simulink model "Missile_Simulink_model"  (R2021a)
settings: Solver=ode4  StartTime=0.0  StopTime=10  FixedStep=Step_Size  RelTol=1e-3  EnableMultiTasking=on
InitFcn:
  | clc ;
  | clear all ;
  | close all ;
  | Missile_Data ;
  | Sim_Parameters ;
values from neighbouring files (symbols this model uses):
  D = 0.150    (= 0.15)    [Missile_Data.m]
  K_A = 0.0270    (= 0.027)    [Missile_Data.m]
  K_DC = 0.8443    [Missile_Data.m]
  K_p = 0.01    [Missile_Data.m]
  K_phi = 20.0    (= 20)    [Missile_Data.m]
  K_R = 0.0777    [Missile_Data.m]
  Mass = 30.0    (= 30)    [Missile_Data.m]
  Omega_i = -6.5208    [Missile_Data.m]
  S = ( pi / 4 ) * D^2    (= 0.0176714586764)    [Missile_Data.m]
  Tbl_ALPHAT = [ 0     4     8    12    16 ]    [Missile_Data.m]
  Tbl_CL_ALPHAT = [ -0.0988   -0.4859   -0.5870   -0.4802   -0.3334   -0.0210 ]    [Missile_Data.m]
  Tbl_CL_DEL_R = [ 5.2712    5.7640    6.1650    6.6234    7.1963    8.4110 ]    [Missile_Data.m]
  Tbl_CL_P = [ -17.9516  -19.6297  -20.9956  -22.5566  -24.5079  -28.6446 ]    [Missile_Data.m]
  Tbl_CM_0 = [ 0   -2.2250   -3.9280   -4.8580   -5.6940 ... (first row only)    [Missile_Data.m]
  Tbl_CM_DEL_P = [ -20.7182  -22.5631  -23.6059  -24.7632  -26.1269  -29.5646 ]    [Missile_Data.m]
  Tbl_CM_PHIT = [ 0   -0.0024   -0.0898   -0.2360   -0.3546 ... (first row only)    [Missile_Data.m]
  Tbl_CM_Q = [ -82.9643  -47.4409  -32.7732  -16.7304  -43.2010  -56.1499 ]    [Missile_Data.m]
  Tbl_CN_DEL_Y = [ -0.3616   -0.3938   -0.4120   -0.4322   -0.4560   -0.5160 ]    [Missile_Data.m]
  Tbl_CN_PHIT = [ 0    0.0040    0.0098    0.1116    0.3049 ... (first row only)    [Missile_Data.m]
  Tbl_CN_R = [ -82.9643  -47.4409  -32.7732  -16.7304  -43.2010  -56.1499 ]    [Missile_Data.m]
  Tbl_CX_0 = [ -0.3840   -0.3670   -0.3550   -0.3460   -0.3390   -0.3410 ]    [Missile_Data.m]
  Tbl_CX_ALPHAT = [ 0.0788    0.0752    0.0680    0.0573    0.0573    0.0573 ]    [Missile_Data.m]
  Tbl_CX_DEL_EFF = [ -16.8080  -17.8585  -18.9090  -19.9595  -20.4847  -23.1110 ]    [Missile_Data.m]
  Tbl_CY_DEL_Y = [ 5.3056    5.7754    6.0504    6.3484    6.6921    7.5745 ]    [Missile_Data.m]
  Tbl_CY_PHIT = [ 0    0.0070    0.0819    0.2313    0.2992 ... (first row only)    [Missile_Data.m]
  Tbl_CZ_0 = [ 0   -2.0680   -3.9700   -5.4250   -6.6810 ... (first row only)    [Missile_Data.m]
  Tbl_CZ_DEL_P = [ -5.3056   -5.7754   -6.0504   -6.3484   -6.6921   -7.5745 ]    [Missile_Data.m]
  Tbl_CZ_PHIT = [ 0    0.0089    0.1842    0.3041    0.2039 ... (first row only)    [Missile_Data.m]
  Tbl_MACH = [ 0.2    0.3    0.4    0.5    0.6    0.7 ]    [Missile_Data.m]
  UNIT_GRAV = 9.81    [Sim_Parameters.m]
  Wn_Act = 25.0 * 2 * pi    (= 157.079632679)    [Missile_Data.m]
  XCG = 0.809    [Missile_Data.m]
  XREF = 0.809    [Missile_Data.m]
  Zeta_Act = 0.707    [Missile_Data.m]
libraries: simulink_extras x6, aerolibtransform2 x4, aerolibasang x3, aerolibconvert2 x2, shared6dof x1, aerolibatmos2 x1
(part 1 of 2)
settings Model: Creator=e803534  LastModifiedBy=s347520
settings SolverCC: AlgebraicLoopSolver=TrustRegion
settings DataIOCC: ReturnWorkspaceOutputs=off
settings OptimizationCC: LifeSpan=inf
settings DebuggingCC: UnconnectedInputMsg=none  UnconnectedOutputMsg=none  UnconnectedLineMsg=none  SFUnexpectedBacktrackingDiag=warning  SFNoUnconditionalDefaultTransitionDiag=warning  SFMachineParentedDataDiag=warning  ArithmeticOperatorsInVariantConditions=warning
settings SFSimCC: SimUseLocalCustomCode=off  CustomCodeUndefinedFunction=UseInterfaceOnly
settings RTWCC: RTWUseLocalCustomCode=off
settings CodeAppCC: StateflowObjectComments=on
settings GRTTargetCC: TargetLangStandard=C89/C90 (ANSI)
settings ConfigComp: CovMetricSettings=dw  CovSaveCumulativeToWorkspaceVar=on  CovSaveSingleToWorkspaceVar=on  CovExternalEMLEnable=off

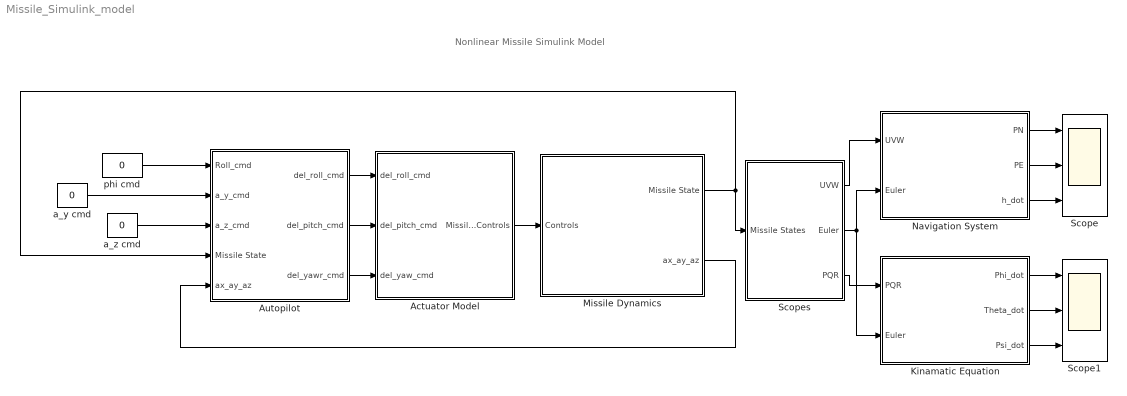
== system Missile_Simulink_model ==
  note: Nonlinear Missile Simulink Model
  Actuator Model : Subsystem
  "Autopilot " : Subsystem
  Kinamatic Equation : Subsystem
  Missile Dynamics : Subsystem
  Navigation System : Subsystem
  Scope : Scope  NumInputPorts=3
  Scope1 : Scope  NumInputPorts=3
  Scopes : Subsystem
  a_y cmd : Constant  Value=0
  a_z cmd : Constant  Value=0
  phi cmd : Constant  Value=0
  wires:
  "Autopilot "/2(del_pitch_cmd) -> Actuator Model/2(del_pitch_cmd)
  "Autopilot "/1(del_roll_cmd) -> Actuator Model/1(del_roll_cmd)
  "Autopilot "/3(del_yawr_cmd) -> Actuator Model/3(del_yaw_cmd)
  Missile Dynamics/1(Missile State) -> "Autopilot "/4(Missile State), Scopes/1(Missile States)
  a_z cmd/1 -> "Autopilot "/3(a_z_cmd)
  phi cmd/1 -> "Autopilot "/1(Roll_cmd)
  a_y cmd/1 -> "Autopilot "/2(a_y_cmd)
  Missile Dynamics/2(ax_ay_az) -> "Autopilot "/5(ax_ay_az)
  Actuator Model/1(Missile_Controls) -> Missile Dynamics/1(Controls)
  Scopes/1(UVW) -> Navigation System/1(UVW)
  Scopes/2(Euler) -> Kinamatic Equation/2(Euler), Navigation System/2(Euler)
  Navigation System/1(PN) -> Scope/1
  Navigation System/2(PE) -> Scope/2
  Navigation System/3(h_dot) -> Scope/3
  Scopes/3(PQR) -> Kinamatic Equation/1(PQR)
  Kinamatic Equation/1(Phi_dot) -> Scope1/1
  Kinamatic Equation/2(Theta_dot) -> Scope1/2
  Kinamatic Equation/3(Psi_dot) -> Scope1/3

== system Missile_Simulink_model/Actuator Model ==
  note: Actuator Model
  del_roll_cmd : Inport
  del_pitch_cmd : Inport  Port=2
  del_yaw_cmd : Inport  Port=3
  Mux : Mux  Inputs=3
  Saturation : Saturate  UpperLimit=10  LowerLimit=-10
  Saturation1 : Saturate  UpperLimit=10  LowerLimit=-10
  Saturation2 : Saturate  UpperLimit=10  LowerLimit=-10
  Transfer Fcn : TransferFcn  Numerator=[Wn_Act^2]  Denominator=[1 2*Zeta_Act*Wn_Act Wn_Act^2]
  Transfer Fcn1 : TransferFcn  Numerator=[Wn_Act^2]  Denominator=[1 2*Zeta_Act*Wn_Act Wn_Act^2]
  Transfer Fcn2 : TransferFcn  Numerator=[Wn_Act^2]  Denominator=[1 2*Zeta_Act*Wn_Act Wn_Act^2]
  Missile_Controls : Outport  VectorParamsAs1DForOutWhenUnconnected=off
  wires:
  del_roll_cmd/1 -> Transfer Fcn/1
  Mux/1 -> Missile_Controls/1
  del_yaw_cmd/1 -> Transfer Fcn2/1
  del_pitch_cmd/1 -> Transfer Fcn1/1
  Transfer Fcn/1 -> Saturation/1
  Transfer Fcn1/1 -> Saturation1/1
  Transfer Fcn2/1 -> Saturation2/1
  Saturation/1 -> Mux/1
  Saturation2/1 -> Mux/3
  Saturation1/1 -> Mux/2

== system Missile_Simulink_model/Autopilot  ==
  note: Autopilot
  Roll_cmd : Inport
  a_y_cmd : Inport  Port=2
  a_z_cmd : Inport  Port=3
  Missile State : Inport  Port=4
  ax_ay_az : Inport  Port=5
  Mux : Mux  Inputs=3
  Pitch Control : Subsystem
  Roll Control : Subsystem
  Scope : Scope
  Yaw Control : Subsystem
  del_roll_cmd : Outport  VectorParamsAs1DForOutWhenUnconnected=off
  del_pitch_cmd : Outport  Port=2  VectorParamsAs1DForOutWhenUnconnected=off
  del_yawr_cmd : Outport  Port=3  VectorParamsAs1DForOutWhenUnconnected=off
  wires:
  Missile State/1 -> Pitch Control/2(Missile_State), Yaw Control/1(Missile_State), Roll Control/2(Missile_State)
  a_z_cmd/1 -> Pitch Control/1(a_z_cmd)
  Pitch Control/1(del_p_cmd) -> Mux/2, del_pitch_cmd/1
  Roll_cmd/1 -> Roll Control/1(Roll_cmd)
  Roll Control/1(del_r_cmd) -> Mux/1, del_roll_cmd/1
  a_y_cmd/1 -> Yaw Control/2("a_y_cmd ")
  Yaw Control/1(del_r_cmd) -> Mux/3, del_yawr_cmd/1
  ax_ay_az/1 -> Pitch Control/3(ax_ay_az), Yaw Control/3(ax_ay_az)
  Mux/1 -> Scope/1

== system Missile_Simulink_model/Kinamatic Equation ==
  PQR : Inport
  Euler : Inport  Port=2
  Demux : Demux  Outputs=3
  Demux2 : Demux  Outputs=3
  MATLAB Function4 : MATLAB Function  TreatAsAtomicUnit=on
  Phi_dot : Outport
  Theta_dot : Outport  Port=2
  Psi_dot : Outport  Port=3
  wires:
  PQR/1 -> Demux2/1
  Euler/1 -> Demux/1
  Demux/1 -> MATLAB Function4/4(phi)
  Demux/2 -> MATLAB Function4/5(theta)
  Demux/3 -> MATLAB Function4/6(psi)
  Demux2/1 -> MATLAB Function4/1(p)
  Demux2/2 -> MATLAB Function4/2(q)
  Demux2/3 -> MATLAB Function4/3(r)
  MATLAB Function4/1(Phi_dot) -> Phi_dot/1
  MATLAB Function4/2(Theta_dot) -> Theta_dot/1
  MATLAB Function4/3(Psi_dot) -> Psi_dot/1

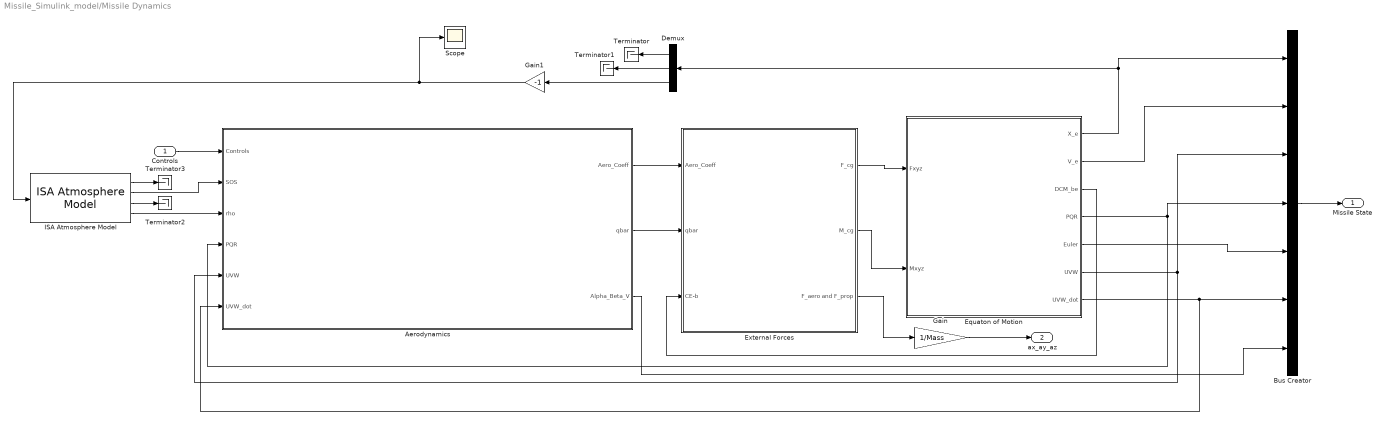
== system Missile_Simulink_model/Missile Dynamics ==
  Controls : Inport
  Aerodynamics : Subsystem
  Bus Creator : BusCreator  Inputs=7
  Demux : Demux  Outputs=3
  Equaton of Motion : Subsystem
  External Forces : Subsystem
  Gain : Gain  Gain=1/Mass
  Gain1 : Gain  Gain=-1
  ISA Atmosphere Model : aerolibatmos2/ISA Atmosphere Model  custom=off  g=9.80665  gamma=1.4  R=287.0531  L=0.0065  h_trop=11000  h_strat=20000  rho0=1.225  P0=101325  T0=288.15  h0=0
  Scope : Scope
  Terminator{,1..3} (4 alike) : Terminator
  Missile State : Outport  VectorParamsAs1DForOutWhenUnconnected=off
  ax_ay_az : Outport  Port=2  VectorParamsAs1DForOutWhenUnconnected=off
  wires:
  Bus Creator/1 -> Missile State/1
  External Forces/3(F_aero and F_prop) -> Gain/1
  Gain/1 -> ax_ay_az/1
  Controls/1 -> Aerodynamics/1(Controls)
  ISA Atmosphere Model/2 -> Aerodynamics/2(SOS)
  ISA Atmosphere Model/4 -> Aerodynamics/3(rho)
  Aerodynamics/1(Aero_Coeff) -> External Forces/1(Aero_Coeff)
  Aerodynamics/2(qbar) -> External Forces/2(qbar)
  Aerodynamics/3(Alpha_Beta_V) -> Bus Creator/7
  Equaton of Motion/4(PQR) -> Aerodynamics/4(PQR), Bus Creator/4
  Equaton of Motion/6(UVW) -> Bus Creator/3, Aerodynamics/5(UVW)
  Equaton of Motion/2(V_e) -> Bus Creator/2
  Equaton of Motion/1(X_e) -> Demux/1, Bus Creator/1
  Equaton of Motion/7(UVW_dot) -> Aerodynamics/6(UVW_dot), Bus Creator/6
  External Forces/1(F_cg) -> Equaton of Motion/1(Fxyz)
  External Forces/2(M_cg) -> Equaton of Motion/2(Mxyz)
  Equaton of Motion/3(DCM_be) -> External Forces/3(CE-b)
  Equaton of Motion/5(Euler) -> Bus Creator/5
  Demux/3 -> Gain1/1
  Gain1/1 -> Scope/1, ISA Atmosphere Model/1
  Demux/1 -> Terminator/1
  Demux/2 -> Terminator1/1
  ISA Atmosphere Model/3 -> Terminator2/1
  ISA Atmosphere Model/1 -> Terminator3/1

== system Missile_Simulink_model/Navigation System ==
  note: h
  note: PE
  note: PN
  note: VD
  note: VE
  note: VN
  UVW : Inport
  Euler : Inport  Port=2
  Demux : Demux  Outputs=3
  Demux1 : Demux  Outputs=3
  Demux2 : Demux  Outputs=3
  Gain : Gain  Gain=-1
  Integrator1 : Integrator
  Integrator2 : Integrator
  Integrator3 : Integrator
  MATLAB Function4 : MATLAB Function  TreatAsAtomicUnit=on
  Matrix Multiply2 : Product  Multiplication=Matrix(*)
  Mux : Mux  Inputs=3
  PN : Outport
  PE : Outport  Port=2
  h_dot : Outport  Port=3
  wires:
  Demux1/2 -> Integrator2/1
  Gain/1 -> Integrator3/1
  Integrator1/1 -> PN/1
  Mux/1 -> Matrix Multiply2/2
  Demux/2 -> MATLAB Function4/2(theta)
  Demux/3 -> MATLAB Function4/3(psi)
  Demux/1 -> MATLAB Function4/1(phi)
  Integrator2/1 -> PE/1
  Integrator3/1 -> h_dot/1
  Demux1/3 -> Gain/1
  Demux1/1 -> Integrator1/1
  Demux2/1 -> Mux/1
  Demux2/2 -> Mux/2
  Demux2/3 -> Mux/3
  Euler/1 -> Demux/1
  UVW/1 -> Demux2/1
  MATLAB Function4/1(C1) -> Matrix Multiply2/1
  Matrix Multiply2/1 -> Demux1/1

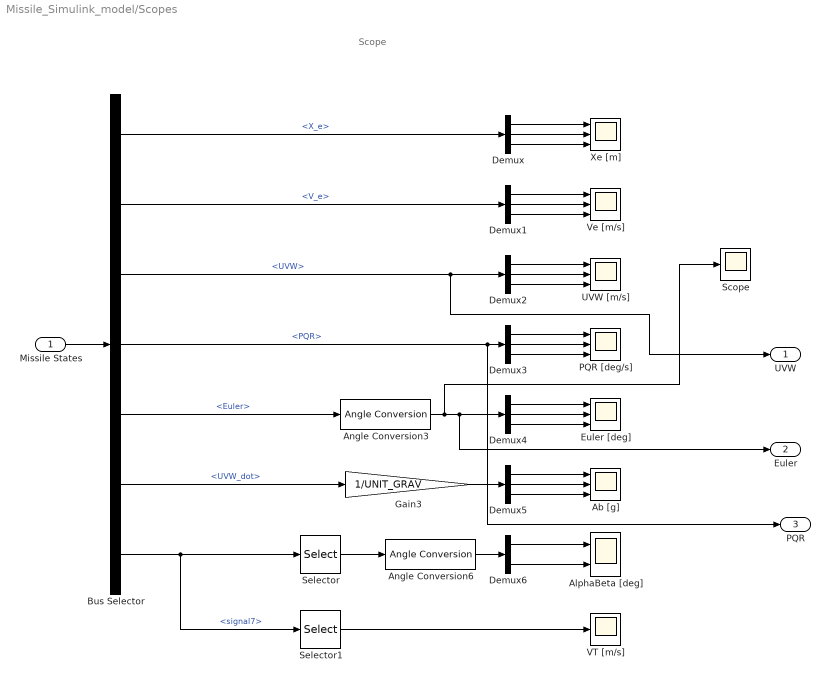
== system Missile_Simulink_model/Scopes ==
  note: Scope
  Missile States : Inport
  Ab [g] : Scope  NumInputPorts=3
  AlphaBeta [deg] : Scope  NumInputPorts=2
  Angle Conversion3 : aerolibconvert2/Angle Conversion  IU=rad  OU=deg
  Angle Conversion6 : aerolibconvert2/Angle Conversion  IU=rad  OU=deg
  Bus Selector : BusSelector  OutputSignals=X_e,V_e,UVW,PQR,Euler,UVW_dot,signal7
  Demux{,1..5} (6 alike) : Demux  Outputs=3
  Demux6 : Demux  Outputs=2
  Euler [deg] : Scope  NumInputPorts=3
  Gain3 : Gain  Gain=1/UNIT_GRAV
  PQR [deg/s] : Scope  NumInputPorts=3
  Scope : Scope
  Selector : Selector  InputPortWidth=3  IndexOptions=Index vector (dialog)  Indices=[1 2]  OutputSizes=1
  Selector1 : Selector  InputPortWidth=3  IndexOptions=Index vector (dialog)  Indices=[3]  OutputSizes=1
  UVW [m/s] : Scope  NumInputPorts=3
  VT [m/s] : Scope
  Ve [m/s] : Scope  NumInputPorts=3
  Xe [m] : Scope  NumInputPorts=3
  UVW : Outport
  Euler : Outport  Port=2
  PQR : Outport  Port=3
  wires:
  Missile States/1 -> Bus Selector/1
  Bus Selector/1 -> Demux/1  "<X_e>"
  Bus Selector/2 -> Demux1/1  "<V_e>"
  Bus Selector/3 -> UVW/1, Demux2/1  "<UVW>"
  Bus Selector/4 -> PQR/1, Demux3/1  "<PQR>"
  Bus Selector/5 -> Angle Conversion3/1  "<Euler>"
  Bus Selector/6 -> Gain3/1  "<UVW_dot>"
  Angle Conversion3/1 -> Scope/1, Euler/1, Demux4/1
  Selector1/1 -> VT [m/s]/1
  Gain3/1 -> Demux5/1
  Demux/1 -> Xe [m]/1
  Demux/2 -> Xe [m]/2
  Demux/3 -> Xe [m]/3
  Demux1/1 -> Ve [m/s]/1
  Demux1/2 -> Ve [m/s]/2
  Demux1/3 -> Ve [m/s]/3
  Demux2/1 -> UVW [m/s]/1
  Demux2/2 -> UVW [m/s]/2
  Demux2/3 -> UVW [m/s]/3
  Demux3/1 -> PQR [deg/s]/1
  Demux3/2 -> PQR [deg/s]/2
  Demux3/3 -> PQR [deg/s]/3
  Demux4/1 -> Euler [deg]/1
  Demux4/2 -> Euler [deg]/2
  Demux4/3 -> Euler [deg]/3
  Demux5/1 -> Ab [g]/1
  Demux5/2 -> Ab [g]/2
  Demux5/3 -> Ab [g]/3
  Demux6/2 -> AlphaBeta [deg]/2
  Demux6/1 -> AlphaBeta [deg]/1
  Angle Conversion6/1 -> Demux6/1
  Bus Selector/7 -> Selector1/1, Selector/1  "<signal7>"
  Selector/1 -> Angle Conversion6/1

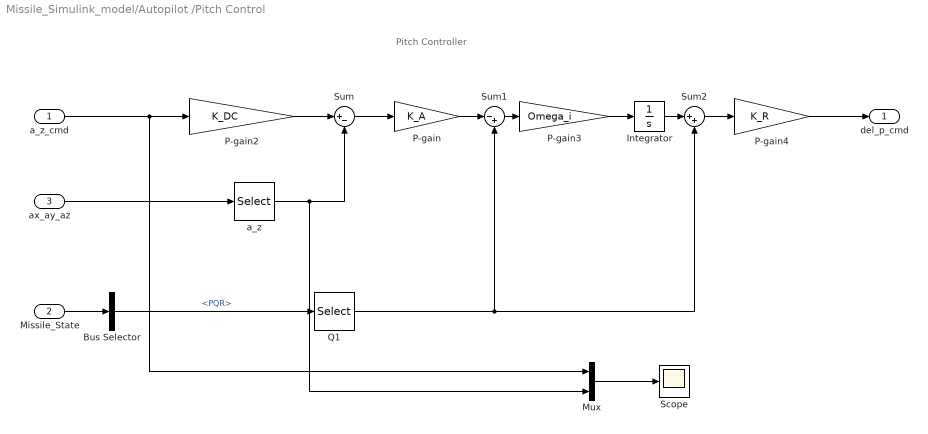
== system Missile_Simulink_model/Autopilot /Pitch Control ==
  note: Pitch Controller
  a_z_cmd : Inport
  Missile_State : Inport  Port=2
  ax_ay_az : Inport  Port=3
  Bus Selector : BusSelector  OutputSignals=PQR
  Integrator : Integrator
  Mux : Mux  Inputs=2
  P-gain : Gain  Gain=K_A
  P-gain2 : Gain  Gain=K_DC
  P-gain3 : Gain  Gain=Omega_i
  P-gain4 : Gain  Gain=K_R
  Q1 : Selector  InputPortWidth=3  IndexOptions=Index vector (dialog)  Indices=[2]  OutputSizes=1
  Scope : Scope
  Sum : Sum  Inputs=|+-
  Sum1 : Sum  Inputs=|-+
  Sum2 : Sum  Inputs=|++
  a_z : Selector  InputPortWidth=3  IndexOptions=Index vector (dialog)  Indices=[3]  OutputSizes=1
  del_p_cmd : Outport  VectorParamsAs1DForOutWhenUnconnected=off
  wires:
  Missile_State/1 -> Bus Selector/1
  P-gain/1 -> Sum1/1
  a_z/1 -> Mux/2, Sum/2
  ax_ay_az/1 -> a_z/1
  P-gain4/1 -> del_p_cmd/1
  Bus Selector/1 -> Q1/1  "<PQR>"
  Q1/1 -> Sum2/2, Sum1/2
  a_z_cmd/1 -> Mux/1, P-gain2/1
  Sum1/1 -> P-gain3/1
  Sum/1 -> P-gain/1
  P-gain2/1 -> Sum/1
  P-gain3/1 -> Integrator/1
  Sum2/1 -> P-gain4/1
  Mux/1 -> Scope/1
  Integrator/1 -> Sum2/1

== system Missile_Simulink_model/Autopilot /Roll Control ==
  note: Roll Controller
  Roll_cmd : Inport
  Missile_State : Inport  Port=2
  Bus Selector : BusSelector  OutputSignals=Euler,PQR
  P : Selector  InputPortWidth=3  IndexOptions=Index vector (dialog)  Indices=[1]  OutputSizes=1
  P-gain2 : Gain  Gain=K_phi
  P-gain3 : Gain  Gain=K_p
  PHI : Selector  InputPortWidth=3  IndexOptions=Index vector (dialog)  Indices=[1]  OutputSizes=1
  Sum : Sum  Inputs=|+-
  Sum2 : Sum  Inputs=|+-
  del_r_cmd : Outport  VectorParamsAs1DForOutWhenUnconnected=off
  wires:
  P-gain2/1 -> Sum2/1
  Missile_State/1 -> Bus Selector/1
  Bus Selector/2 -> P/1  "<PQR>"
  P/1 -> Sum2/2
  PHI/1 -> Sum/2
  Roll_cmd/1 -> Sum/1
  Sum2/1 -> P-gain3/1
  Sum/1 -> P-gain2/1
  Bus Selector/1 -> PHI/1  "<Euler>"
  P-gain3/1 -> del_r_cmd/1

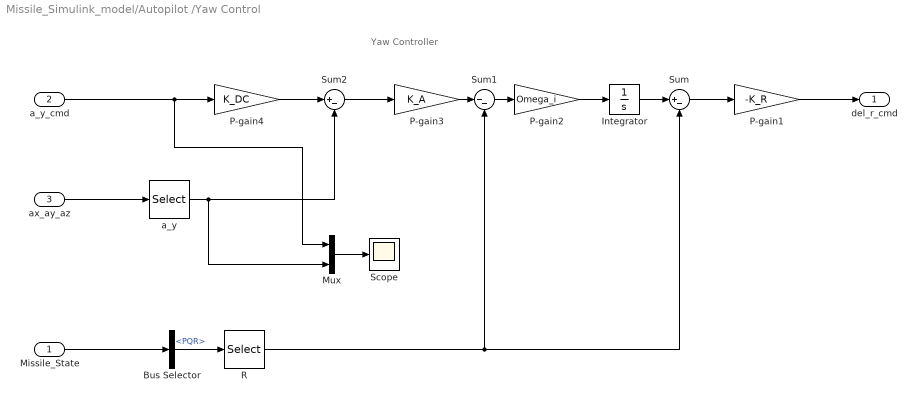
== system Missile_Simulink_model/Autopilot /Yaw Control ==
  note: Yaw Controller
  Missile_State : Inport
  "a_y_cmd " : Inport  Port=2
  ax_ay_az : Inport  Port=3
  Bus Selector : BusSelector  OutputSignals=PQR
  Integrator : Integrator
  Mux : Mux  Inputs=2
  P-gain1 : Gain  Gain=-K_R
  P-gain2 : Gain  Gain=Omega_i
  P-gain3 : Gain  Gain=K_A
  P-gain4 : Gain  Gain=K_DC
  R : Selector  InputPortWidth=3  IndexOptions=Index vector (dialog)  Indices=[3]  OutputSizes=1
  Scope : Scope
  Sum : Sum  Inputs=|+-
  Sum1 : Sum  Inputs=|--
  Sum2 : Sum  Inputs=|+-
  a_y : Selector  InputPortWidth=3  IndexOptions=Index vector (dialog)  Indices=[2]  OutputSizes=1
  del_r_cmd : Outport  VectorParamsAs1DForOutWhenUnconnected=off
  wires:
  ax_ay_az/1 -> a_y/1
  P-gain3/1 -> Sum1/1
  R/1 -> Sum1/2, Sum/2
  Sum2/1 -> P-gain3/1
  P-gain1/1 -> del_r_cmd/1
  Sum1/1 -> P-gain2/1
  Bus Selector/1 -> R/1  "<PQR>"
  "a_y_cmd "/1 -> Mux/1, P-gain4/1
  Sum/1 -> P-gain1/1
  Integrator/1 -> Sum/1
  Missile_State/1 -> Bus Selector/1
  P-gain2/1 -> Integrator/1
  a_y/1 -> Mux/2, Sum2/2
  Mux/1 -> Scope/1
  P-gain4/1 -> Sum2/1

== system Missile_Simulink_model/Missile Dynamics/Aerodynamics ==
  Controls : Inport
  SOS : Inport  Port=2
  rho : Inport  Port=3
  PQR : Inport  Port=4
  UVW : Inport  Port=5
  UVW_dot : Inport  Port=6
  Aerodynamic Coefficient : Subsystem
  Ground : Ground
  Ground1 : Ground
  Wind-axes Velocitie : Subsystem  AncestorBlock=UAS_Model_library/External Forces/Aerodynamics/Wind-axes Velocitie
  Aero_Coeff : Outport  VectorParamsAs1DForOutWhenUnconnected=off
  qbar : Outport  Port=2  VectorParamsAs1DForOutWhenUnconnected=off
  Alpha_Beta_V : Outport  Port=3  VectorParamsAs1DForOutWhenUnconnected=off
  wires:
  rho/1 -> Wind-axes Velocitie/4(Rho)
  UVW/1 -> Wind-axes Velocitie/1(UVW)
  Wind-axes Velocitie/1(Alpha_Beta_V) -> Alpha_Beta_V/1, Aerodynamic Coefficient/3(Alpha_Beta_V1), Aerodynamic Coefficient/2(Alpha_Beta_V)
  Wind-axes Velocitie/2(Mach) -> Aerodynamic Coefficient/4(Mach Number)
  Ground1/1 -> Wind-axes Velocitie/2(Wind_Vel)
  Ground/1 -> Wind-axes Velocitie/7(Wind_Rate)
  Controls/1 -> Aerodynamic Coefficient/1(Control)
  PQR/1 -> Aerodynamic Coefficient/5(PQR), Wind-axes Velocitie/6(PQR)
  Wind-axes Velocitie/3(qbar) -> qbar/1
  UVW_dot/1 -> Wind-axes Velocitie/5(UVW_dot)
  Aerodynamic Coefficient/1(Aero_Coeff) -> Aero_Coeff/1
  SOS/1 -> Wind-axes Velocitie/3(SoS)

== system Missile_Simulink_model/Missile Dynamics/Equaton of Motion ==
  Fxyz : Inport
  Mxyz : Inport  Port=2
  Equation of mortion : Subsystem
  Terminator2 : Terminator
  X_e : Outport  VectorParamsAs1DForOutWhenUnconnected=off
  V_e : Outport  Port=2  VectorParamsAs1DForOutWhenUnconnected=off
  DCM_be : Outport  Port=3  VectorParamsAs1DForOutWhenUnconnected=off
  PQR : Outport  Port=4  VectorParamsAs1DForOutWhenUnconnected=off
  Euler : Outport  Port=5  VectorParamsAs1DForOutWhenUnconnected=off
  UVW : Outport  Port=6  VectorParamsAs1DForOutWhenUnconnected=off
  UVW_dot : Outport  Port=7  VectorParamsAs1DForOutWhenUnconnected=off
  wires:
  Fxyz/1 -> Equation of mortion/1(Forces)
  Mxyz/1 -> Equation of mortion/2(Moments)
  Equation of mortion/1(V_e) -> V_e/1
  Equation of mortion/2(X_e) -> X_e/1
  Equation of mortion/3(Euler) -> Euler/1
  Equation of mortion/4(DCM) -> DCM_be/1
  Equation of mortion/5(UVW) -> UVW/1
  Equation of mortion/6(PQR) -> PQR/1
  Equation of mortion/7(pdot,qdot,rdot) -> Terminator2/1
  Equation of mortion/8(UVW_dot) -> UVW_dot/1

== system Missile_Simulink_model/Missile Dynamics/External Forces ==
  Aero_Coeff : Inport
  qbar : Inport  Port=2
  CE-b : Inport  Port=3
  Add : Sum
  Aerodynamic Force & Moment : Subsystem  AncestorBlock=UAS_Model_library/External Forces/Aerodynamics/Aerodynamic Force & Moment
  Propulsive Force & Moment : Subsystem  AncestorBlock=UAS_Model_library/External Forces/Propulsive/Propulsive Force & Moment
  Total Force & Moment : Subsystem  AncestorBlock=UAS_Model_library/External Forces/Total Force & Moment
  F_cg : Outport  VectorParamsAs1DForOutWhenUnconnected=off
  M_cg : Outport  Port=2  VectorParamsAs1DForOutWhenUnconnected=off
  F_aero and F_prop : Outport  Port=3  VectorParamsAs1DForOutWhenUnconnected=off
  wires:
  Total Force & Moment/2(M_cg) -> M_cg/1
  Aerodynamic Force & Moment/2(M_aero) -> Total Force & Moment/2(M_aero)
  Propulsive Force & Moment/2(M_prop) -> Total Force & Moment/4(M_prop)
  Total Force & Moment/1(F_cg) -> F_cg/1
  Aerodynamic Force & Moment/1(F_aero) -> Add/1, Total Force & Moment/1(F_aero)
  Propulsive Force & Moment/1(F_prop) -> Add/2, Total Force & Moment/3(F_prop)
  qbar/1 -> Aerodynamic Force & Moment/2(qbar)
  Aero_Coeff/1 -> Aerodynamic Force & Moment/1(Aero_Coeff)
  Add/1 -> F_aero and F_prop/1
  CE-b/1 -> Total Force & Moment/5("cE-B ")

== system Missile_Simulink_model/Missile Dynamics/Aerodynamics/Aerodynamic Coefficient ==
  Control : Inport
  Alpha_Beta_V : Inport  Port=2
  Alpha_Beta_V1 : Inport  Port=3
  Mach Number : Inport  Port=4
  PQR : Inport  Port=5
  Aerodynamics : Subsystem
  delta_eff : Subsystem
  total angle of AoA and Roll : Subsystem
  Aero_Coeff : Outport  VectorParamsAs1DForOutWhenUnconnected=off
  wires:
  total angle of AoA and Roll/1(alpha_t) -> Aerodynamics/4(alpha_t)
  Alpha_Beta_V/1 -> Aerodynamics/6(alpha_beta_V)
  total angle of AoA and Roll/2(phi_t) -> Aerodynamics/5(phi_t)
  delta_eff/1(delta_eff) -> Aerodynamics/2(delta_eff)
  Control/1 -> Aerodynamics/3(control inputs), delta_eff/1(controll)
  Aerodynamics/1(Aero_Coeff) -> Aero_Coeff/1
  Alpha_Beta_V1/1 -> total angle of AoA and Roll/1(alpha_beta_V)
  Mach Number/1 -> Aerodynamics/1(Mach Number)
  PQR/1 -> Aerodynamics/7(PQR)

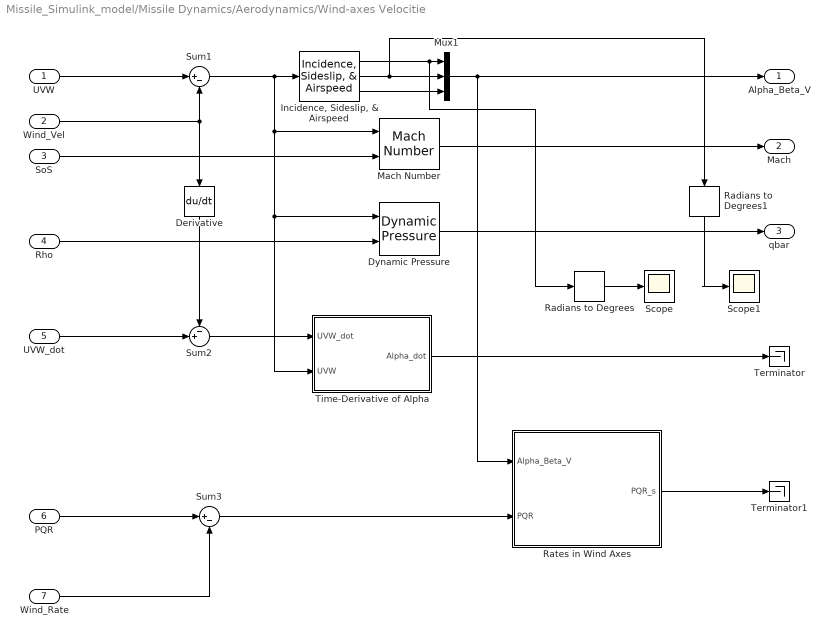
== system Missile_Simulink_model/Missile Dynamics/Aerodynamics/Wind-axes Velocitie ==
  UVW : Inport
  Wind_Vel : Inport  Port=2
  SoS : Inport  Port=3
  Rho : Inport  Port=4
  UVW_dot : Inport  Port=5
  PQR : Inport  Port=6
  Wind_Rate : Inport  Port=7
  Derivative : Derivative
  Dynamic Pressure : aerolibasang/Dynamic Pressure
  "Incidence, Sideslip, & Airspeed" : aerolibasang/Incidence, Sideslip, & Airspeed
  Mach Number : aerolibasang/Mach Number
      settings: SourceProductBaseCode=AE
  Mux1 : Mux  Inputs=3
  Radians to Degrees : simulink_extras/Transformations/Radians to Degrees
  Radians to Degrees1 : simulink_extras/Transformations/Radians to Degrees
  Rates in Wind Axes : Subsystem
  Scope : Scope
  Scope1 : Scope
  Sum1 : Sum  Inputs=|+-  InputSameDT=on  SaturateOnIntegerOverflow=on  OutDataTypeStr=Inherit: Same as first input
  Sum2 : Sum  Inputs=-+|  InputSameDT=on  SaturateOnIntegerOverflow=on  OutDataTypeStr=Inherit: Same as first input
  Sum3 : Sum  Inputs=|+-  InputSameDT=on  SaturateOnIntegerOverflow=on  OutDataTypeStr=Inherit: Same as first input
  Terminator : Terminator
  Terminator1 : Terminator
  Time-Derivative of Alpha : Subsystem
  Alpha_Beta_V : Outport  VectorParamsAs1DForOutWhenUnconnected=off
  Mach : Outport  Port=2  VectorParamsAs1DForOutWhenUnconnected=off
  qbar : Outport  Port=3  VectorParamsAs1DForOutWhenUnconnected=off
  wires:
  Wind_Rate/1 -> Sum3/2
  PQR/1 -> Sum3/1
  Sum3/1 -> Rates in Wind Axes/2(PQR)
  Rates in Wind Axes/1(PQR_s) -> Terminator1/1
  "Incidence, Sideslip, & Airspeed"/3 -> Mux1/3
  "Incidence, Sideslip, & Airspeed"/2 -> Radians to Degrees1/1, Mux1/2
  "Incidence, Sideslip, & Airspeed"/1 -> Radians to Degrees/1, Mux1/1
  Sum1/1 -> "Incidence, Sideslip, & Airspeed"/1, Mach Number/1, Dynamic Pressure/1, Time-Derivative of Alpha/2(UVW)
  Mux1/1 -> Alpha_Beta_V/1, Rates in Wind Axes/1(Alpha_Beta_V)
  UVW/1 -> Sum1/1
  Wind_Vel/1 -> Derivative/1, Sum1/2
  Mach Number/1 -> Mach/1
  SoS/1 -> Mach Number/2
  Rho/1 -> Dynamic Pressure/2
  Dynamic Pressure/1 -> qbar/1
  Time-Derivative of Alpha/1(Alpha_dot) -> Terminator/1
  UVW_dot/1 -> Sum2/2
  Sum2/1 -> Time-Derivative of Alpha/1(UVW_dot)
  Derivative/1 -> Sum2/1
  Radians to Degrees/1 -> Scope/1
  Radians to Degrees1/1 -> Scope1/1

== system Missile_Simulink_model/Missile Dynamics/Equaton of Motion/Equation of mortion ==
  Forces : Inport
  Moments : Inport  Port=2
  6DOF (Euler Angles) : shared6dof/6DOF (Euler Angles)  units=Metric (MKS)  mtype=Fixed  rep=Euler Angles  xme_0=Init_Pos  Vm_0=Init_Vel  eul_0=Init_Euler  pm_0=Init_Rate  mass_0=Mass  mass_e=0.5  mass_f=2.0  inertia=I_TENSOR  inertia_e=eye(3)  inertia_f=2*eye(3)  k_quat=1.0  vre_flag=on  abi_flag=off  aMode=0  xme_statename=''  Vm_statename=''  eul_statename=''  quat_statename=''  pm_statename=''  mass_statename=''
      settings: SourceProductBaseCode=AE,PW,DR,MT,UV,VE
  V_e : Outport
  X_e : Outport  Port=2
  Euler : Outport  Port=3
  DCM : Outport  Port=4
  UVW : Outport  Port=5
  PQR : Outport  Port=6
  pdot,qdot,rdot : Outport  Port=7
  UVW_dot : Outport  Port=8
  wires:
  6DOF (Euler Angles)/1 -> V_e/1  "V_e"
  6DOF (Euler Angles)/6 -> PQR/1  "PQR"
  6DOF (Euler Angles)/3 -> Euler/1  "Euler"
  6DOF (Euler Angles)/2 -> X_e/1  "X_e"
  6DOF (Euler Angles)/7 -> pdot,qdot,rdot/1
  Forces/1 -> 6DOF (Euler Angles)/1
  6DOF (Euler Angles)/8 -> UVW_dot/1  "UVW_dot"
  Moments/1 -> 6DOF (Euler Angles)/2
  6DOF (Euler Angles)/4 -> DCM/1
  6DOF (Euler Angles)/5 -> UVW/1  "UVW"

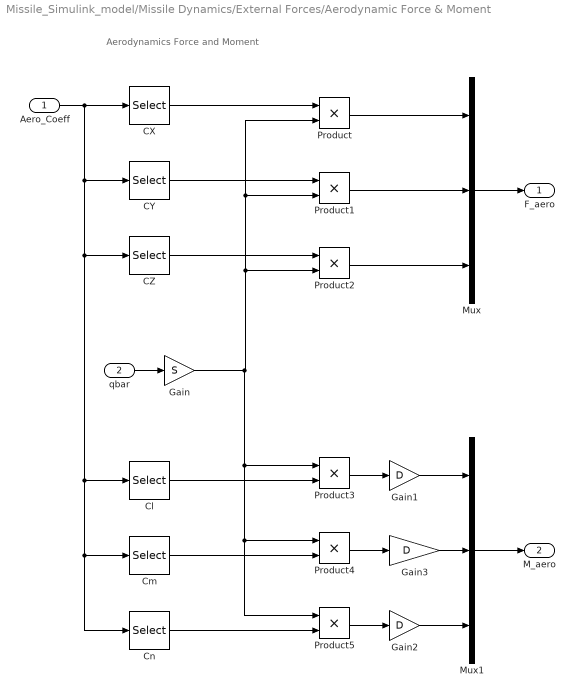
== system Missile_Simulink_model/Missile Dynamics/External Forces/Aerodynamic Force & Moment ==
  note: Aerodynamics Force and Moment
  Aero_Coeff : Inport
  qbar : Inport  Port=2
  CX : Selector  InputPortWidth=6  IndexOptions=Index vector (dialog)  Indices=[1]  OutputSizes=1
  CY : Selector  InputPortWidth=6  IndexOptions=Index vector (dialog)  Indices=[2]  OutputSizes=1
  CZ : Selector  InputPortWidth=6  IndexOptions=Index vector (dialog)  Indices=[3]  OutputSizes=1
  Cl : Selector  InputPortWidth=6  IndexOptions=Index vector (dialog)  Indices=[4]  OutputSizes=1
  Cm : Selector  InputPortWidth=6  IndexOptions=Index vector (dialog)  Indices=[5]  OutputSizes=1
  Cn : Selector  InputPortWidth=6  IndexOptions=Index vector (dialog)  Indices=[6]  OutputSizes=1
  Gain : Gain  Gain=S
  Gain1 : Gain  Gain=D
  Gain2 : Gain  Gain=D
  Gain3 : Gain  Gain=D
  Mux : Mux  Inputs=3
  Mux1 : Mux  Inputs=3
  Product{,1..5} (6 alike) : Product
  F_aero : Outport  VectorParamsAs1DForOutWhenUnconnected=off
  M_aero : Outport  Port=2  VectorParamsAs1DForOutWhenUnconnected=off
  wires:
  Gain3/1 -> Mux1/2
  Gain2/1 -> Mux1/3
  Gain1/1 -> Mux1/1
  Mux1/1 -> M_aero/1
  Product5/1 -> Gain2/1
  Product4/1 -> Gain3/1
  Product3/1 -> Gain1/1
  Cn/1 -> Product5/2
  Cm/1 -> Product4/2
  Cl/1 -> Product3/2
  Mux/1 -> F_aero/1
  Product2/1 -> Mux/3
  Product1/1 -> Mux/2
  Product/1 -> Mux/1
  CZ/1 -> Product2/1
  CY/1 -> Product1/1
  Gain/1 -> Product/2, Product1/2, Product2/2, Product3/1, Product4/1, Product5/1
  CX/1 -> Product/1
  qbar/1 -> Gain/1
  Aero_Coeff/1 -> CX/1, CY/1, CZ/1, Cm/1, Cn/1, Cl/1

== system Missile_Simulink_model/Missile Dynamics/External Forces/Propulsive Force & Moment ==
  note: Propulsive Force and Moment
  Constant : Constant  Value=0
  Mux : Mux  Inputs=3
  Mux1 : Mux  Inputs=3
  Thrust : Constant  Value=0
  F_prop : Outport  VectorParamsAs1DForOutWhenUnconnected=off
  M_prop : Outport  Port=2  VectorParamsAs1DForOutWhenUnconnected=off
  wires:
  Mux/1 -> F_prop/1
  Constant/1 -> Mux/2, Mux1/1, Mux1/2, Mux1/3, Mux/3
  Mux1/1 -> M_prop/1
  Thrust/1 -> Mux/1

== system Missile_Simulink_model/Missile Dynamics/External Forces/Total Force & Moment ==
  note: Total Force and Moment
  F_aero : Inport  PortDimensions=3
  M_aero : Inport  Port=2  PortDimensions=3
  F_prop : Inport  Port=3  PortDimensions=3
  M_prop : Inport  Port=4  PortDimensions=3
  "cE-B " : Inport  Port=5
  Constant : Constant  Value=0
  Gravity : Subsystem  AncestorBlock=UAS_Model_library/Envrionment/Gravity
  Total Force : Sum  Inputs=+++  InputSameDT=on  SaturateOnIntegerOverflow=on  OutDataTypeStr=Inherit: Same as first input
  Total Moment : Sum  Inputs=+++  InputSameDT=on  SaturateOnIntegerOverflow=on  OutDataTypeStr=Inherit: Same as first input
  F_cg : Outport  VectorParamsAs1DForOutWhenUnconnected=off
  M_cg : Outport  Port=2  VectorParamsAs1DForOutWhenUnconnected=off
  wires:
  Gravity/1(Gravity) -> Total Force/3
  Total Moment/1 -> M_cg/1
  M_prop/1 -> Total Moment/3
  F_prop/1 -> Total Force/2
  F_aero/1 -> Total Force/1
  Constant/1 -> Total Moment/1
  M_aero/1 -> Total Moment/2
  "cE-B "/1 -> Gravity/1(cE_B)
  Total Force/1 -> F_cg/1

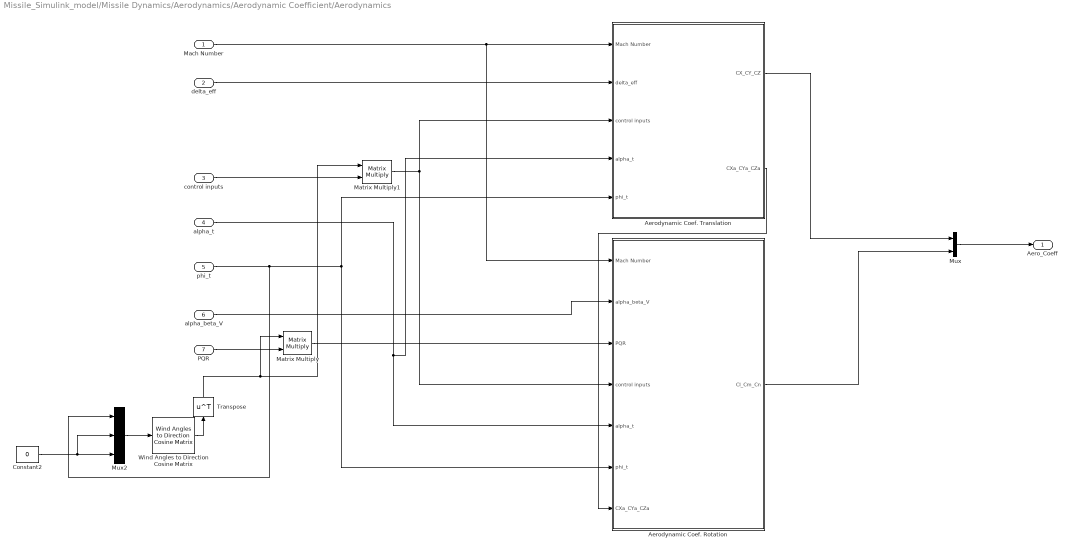
== system Missile_Simulink_model/Missile Dynamics/Aerodynamics/Aerodynamic Coefficient/Aerodynamics ==
  Mach Number : Inport
  delta_eff : Inport  Port=2
  control inputs : Inport  Port=3
  alpha_t : Inport  Port=4
  phi_t : Inport  Port=5
  alpha_beta_V : Inport  Port=6
  PQR : Inport  Port=7
  Aerodynamic Coef. Rotation : Subsystem
  Aerodynamic Coef. Translation : Subsystem
  Constant2 : Constant  Value=0
  Matrix Multiply : Product  Multiplication=Matrix(*)
  Matrix Multiply1 : Product  Multiplication=Matrix(*)
  Mux : Mux  Inputs=2
  Mux2 : Mux  Inputs=3
  Transpose : Math  Operator=transpose  SignedPower=on  SaturateOnIntegerOverflow=on
  Wind Angles to Direction Cosine Matrix : aerolibtransform2/Wind Angles to  Direction Cosine Matrix
      settings: SourceProductBaseCode=AE
  Aero_Coeff : Outport  VectorParamsAs1DForOutWhenUnconnected=off
  wires:
  Aerodynamic Coef. Translation/2(CXa_CYa_CZa) -> Aerodynamic Coef. Rotation/7(CXa_CYa_CZa)
  Mach Number/1 -> Aerodynamic Coef. Rotation/1(Mach Number), Aerodynamic Coef. Translation/1(Mach Number)
  delta_eff/1 -> Aerodynamic Coef. Translation/2(delta_eff)
  Matrix Multiply1/1 -> Aerodynamic Coef. Rotation/4(control inputs), Aerodynamic Coef. Translation/3(control inputs)
  alpha_beta_V/1 -> Aerodynamic Coef. Rotation/2(alpha_beta_V)
  Matrix Multiply/1 -> Aerodynamic Coef. Rotation/3(PQR)
  Aerodynamic Coef. Translation/1(CX_CY_CZ) -> Mux/1
  Mux/1 -> Aero_Coeff/1
  alpha_t/1 -> Aerodynamic Coef. Rotation/5(alpha_t), Aerodynamic Coef. Translation/4(alpha_t)
  phi_t/1 -> Mux2/1, Aerodynamic Coef. Rotation/6(phi_t), Aerodynamic Coef. Translation/5(phi_t)
  Mux2/1 -> Wind Angles to Direction Cosine Matrix/1
  Constant2/1 -> Mux2/2, Mux2/3
  control inputs/1 -> Matrix Multiply1/2
  Wind Angles to Direction Cosine Matrix/1 -> Transpose/1
  PQR/1 -> Matrix Multiply/2
  Transpose/1 -> Matrix Multiply1/1, Matrix Multiply/1
  Aerodynamic Coef. Rotation/1(Cl_Cm_Cn) -> Mux/2

== system Missile_Simulink_model/Missile Dynamics/Aerodynamics/Aerodynamic Coefficient/delta_eff ==
  controll : Inport
  Abs : Abs
  Abs1 : Abs
  Constant : Constant  Value=2
  Divide : Product  Inputs=*/  RndMeth=Zero  SaturateOnIntegerOverflow=on
  Selector : Selector  InputPortWidth=3  IndexOptions=Index vector (dialog)  Indices=[3]  OutputSizes=1
  Selector1 : Selector  InputPortWidth=3  IndexOptions=Index vector (dialog)  Indices=[2]  OutputSizes=1
  Sum : Sum  Inputs=|++
  delta_eff : Outport  VectorParamsAs1DForOutWhenUnconnected=off
  wires:
  Selector1/1 -> Abs1/1
  Sum/1 -> Divide/1
  Constant/1 -> Divide/2
  Divide/1 -> delta_eff/1
  controll/1 -> Selector/1, Selector1/1
  Selector/1 -> Abs/1
  Abs/1 -> Sum/1
  Abs1/1 -> Sum/2

== system Missile_Simulink_model/Missile Dynamics/Aerodynamics/Aerodynamic Coefficient/total angle of AoA and Roll ==
  alpha_beta_V : Inport
  Asin : Trigonometry  Operator=acos
  Atan2 : Trigonometry  Operator=atan2
  Cos : Trigonometry  Operator=cos
  Cos1 : Trigonometry  Operator=cos
  Multiply : Product
  Selector : Selector  InputPortWidth=3  IndexOptions=Index vector (dialog)  Indices=[1]  OutputSizes=1
  Selector1 : Selector  InputPortWidth=3  IndexOptions=Index vector (dialog)  Indices=[2]  OutputSizes=1
  Sin : Trigonometry
  Tan : Trigonometry  Operator=tan
  alpha_t : Outport  VectorParamsAs1DForOutWhenUnconnected=off
  phi_t : Outport  Port=2  VectorParamsAs1DForOutWhenUnconnected=off
  wires:
  Sin/1 -> Atan2/2
  Tan/1 -> Atan2/1
  Selector/1 -> Sin/1, Cos/1
  Selector1/1 -> Tan/1, Cos1/1
  Cos1/1 -> Multiply/2
  Multiply/1 -> Asin/1
  Cos/1 -> Multiply/1
  Atan2/1 -> phi_t/1
  Asin/1 -> alpha_t/1
  alpha_beta_V/1 -> Selector1/1, Selector/1

== system Missile_Simulink_model/Missile Dynamics/Aerodynamics/Wind-axes Velocitie/Rates in Wind Axes ==
  note: Rates in Wind Axes
  Alpha_Beta_V : Inport
  PQR : Inport  Port=2
  Alpha : Selector  InputPortWidth=3  IndexOptions=Index vector (dialog)  Indices=[1]  OutputSizes=1
  Beta_Ref : Constant  Value=0
  Direction Cosine Matrix Body to Wind : aerolibtransform2/Direction Cosine Matrix Body to Wind
      settings: SourceProductBaseCode=AE
  Mux : Mux  Inputs=2
  transform to body axes : Product  Inputs=**  Multiplication=Matrix(*)  InputSameDT=on  SaturateOnIntegerOverflow=on  OutDataTypeStr=Inherit: Same as first input
  PQR_s : Outport  VectorParamsAs1DForOutWhenUnconnected=off
  wires:
  Beta_Ref/1 -> Mux/2
  Mux/1 -> Direction Cosine Matrix Body to Wind/1
  transform to body axes/1 -> PQR_s/1
  PQR/1 -> transform to body axes/2
  Direction Cosine Matrix Body to Wind/1 -> transform to body axes/1  "cB_W"
  Alpha/1 -> Mux/1
  Alpha_Beta_V/1 -> Alpha/1

== system Missile_Simulink_model/Missile Dynamics/Aerodynamics/Wind-axes Velocitie/Time-Derivative of Alpha ==
  note: Time Derivative of Alpha
  UVW_dot : Inport
  UVW : Inport  Port=2
  Add : Sum  Inputs=-+
  Add1 : Sum
  Demux2 : Demux  Outputs=3
  Demux3 : Demux  Outputs=3
  Divide : Product  Inputs=*/
  Math Function2 : Math  Operator=square  SignedPower=on  SaturateOnIntegerOverflow=on
  Math Function3 : Math  Operator=square  SignedPower=on  SaturateOnIntegerOverflow=on
  Product3 : Product
  Product4 : Product
  Terminator2 : Terminator
  Terminator3 : Terminator
  Alpha_dot : Outport  VectorParamsAs1DForOutWhenUnconnected=off
  wires:
  Divide/1 -> Alpha_dot/1
  Add1/1 -> Divide/2
  Math Function3/1 -> Add1/2
  Math Function2/1 -> Add1/1
  Add/1 -> Divide/1
  Product3/1 -> Add/1
  Product4/1 -> Add/2
  Demux3/1 -> Product4/2, Math Function2/1
  Demux2/3 -> Product4/1
  Demux3/3 -> Product3/2, Math Function3/1
  Demux3/2 -> Terminator3/1
  UVW/1 -> Demux3/1
  Demux2/1 -> Product3/1
  Demux2/2 -> Terminator2/1
  UVW_dot/1 -> Demux2/1

== system Missile_Simulink_model/Missile Dynamics/External Forces/Total Force & Moment/Gravity ==
  cE_B : Inport
  Constant : Constant  Value=0
  Constant1 : Constant  Value=Mass
  Display : Display
  Display1 : Display
  "Gravity vector in body frame " : Product  Multiplication=Matrix(*)  InputSameDT=on  SaturateOnIntegerOverflow=on  OutDataTypeStr=Inherit: Same as first input
  Mux1 : Mux  Inputs=3
  g : Gain  Gain=UNIT_GRAV
  Gravity : Outport  VectorParamsAs1DForOutWhenUnconnected=off
  wires:
  Constant1/1 -> g/1
  "Gravity vector in body frame "/1 -> Display/1, Gravity/1
  g/1 -> Mux1/3
  Mux1/1 -> "Gravity vector in body frame "/2
  cE_B/1 -> Display1/1, "Gravity vector in body frame "/1
  Constant/1 -> Mux1/1, Mux1/2

== system Missile_Simulink_model/Missile Dynamics/Aerodynamics/Aerodynamic Coefficient/Aerodynamics/Aerodynamic Coef. Rotation ==
  Mach Number : Inport
  alpha_beta_V : Inport  Port=2
  PQR : Inport  Port=3
  control inputs : Inport  Port=4
  alpha_t : Inport  Port=5
  phi_t : Inport  Port=6
  CXa_CYa_CZa : Inport  Port=7
  Constant2 : Constant  Value=0
  Matrix Multiply : Product  Multiplication=Matrix(*)
  Mux : Mux  Inputs=3
  Mux2 : Mux  Inputs=3
  Subsystem Aero. Coef. Rotation : Subsystem
  Wind Angles to Direction Cosine Matrix : aerolibtransform2/Wind Angles to  Direction Cosine Matrix
      settings: SourceProductBaseCode=AE
  Cl_Cm_Cn : Outport  VectorParamsAs1DForOutWhenUnconnected=off
  wires:
  Mux/1 -> Matrix Multiply/2
  Matrix Multiply/1 -> Cl_Cm_Cn/1
  Mach Number/1 -> Subsystem Aero. Coef. Rotation/1(Mach Number)
  alpha_beta_V/1 -> Subsystem Aero. Coef. Rotation/4(alpha_beta_V)
  PQR/1 -> Subsystem Aero. Coef. Rotation/5(PQR)
  control inputs/1 -> Subsystem Aero. Coef. Rotation/6(control)
  alpha_t/1 -> Subsystem Aero. Coef. Rotation/2(alpha_t)
  phi_t/1 -> Mux2/1, Subsystem Aero. Coef. Rotation/3(phi_t)
  CXa_CYa_CZa/1 -> Subsystem Aero. Coef. Rotation/7(C_X_C_Y_CZ)
  Mux2/1 -> Wind Angles to Direction Cosine Matrix/1
  Constant2/1 -> Mux2/2, Mux2/3
  Wind Angles to Direction Cosine Matrix/1 -> Matrix Multiply/1
  Subsystem Aero. Coef. Rotation/1(C_L_A) -> Mux/1
  Subsystem Aero. Coef. Rotation/2(C_M_A) -> Mux/2
  Subsystem Aero. Coef. Rotation/3(C_N_A) -> Mux/3

== system Missile_Simulink_model/Missile Dynamics/Aerodynamics/Aerodynamic Coefficient/Aerodynamics/Aerodynamic Coef. Translation ==
  Mach Number : Inport
  delta_eff : Inport  Port=2
  control inputs : Inport  Port=3
  alpha_t : Inport  Port=4
  phi_t : Inport  Port=5
  Constant2 : Constant  Value=0
  Matrix Multiply : Product  Multiplication=Matrix(*)
  Mux : Mux  Inputs=3
  Mux2 : Mux  Inputs=3
  Scope : Scope
  Subsystem Aero. Coef. Translation : Subsystem
  Wind Angles to Direction Cosine Matrix : aerolibtransform2/Wind Angles to  Direction Cosine Matrix
      settings: SourceProductBaseCode=AE
  CX_CY_CZ : Outport  VectorParamsAs1DForOutWhenUnconnected=off
  CXa_CYa_CZa : Outport  Port=2  VectorParamsAs1DForOutWhenUnconnected=off
  wires:
  Mux/1 -> Matrix Multiply/2, CXa_CYa_CZa/1
  Matrix Multiply/1 -> CX_CY_CZ/1
  Mux2/1 -> Wind Angles to Direction Cosine Matrix/1
  phi_t/1 -> Mux2/1, Subsystem Aero. Coef. Translation/5(phi_t)
  Constant2/1 -> Mux2/2, Mux2/3
  Mach Number/1 -> Subsystem Aero. Coef. Translation/1(Mach number)
  control inputs/1 -> Subsystem Aero. Coef. Translation/4(control)
  alpha_t/1 -> Subsystem Aero. Coef. Translation/2(alpha_t)
  delta_eff/1 -> Subsystem Aero. Coef. Translation/3(delta_eff)
  Subsystem Aero. Coef. Translation/1(C_X_A) -> Scope/1, Mux/1
  Subsystem Aero. Coef. Translation/2(C_Y_A) -> Mux/2
  Subsystem Aero. Coef. Translation/3(C_Z_A) -> Mux/3
  Wind Angles to Direction Cosine Matrix/1 -> Matrix Multiply/1

== system Missile_Simulink_model/Missile Dynamics/Aerodynamics/Aerodynamic Coefficient/Aerodynamics/Aerodynamic Coef. Rotation/Subsystem Aero. Coef. Rotation ==
  Mach Number : Inport
  alpha_t : Inport  Port=2
  phi_t : Inport  Port=3
  alpha_beta_V : Inport  Port=4
  PQR : Inport  Port=5
  control : Inport  Port=6
  C_X_C_Y_CZ : Inport  Port=7
  "Subsystem C_L_A " : Subsystem
  "Subsystem C_M_A " : Subsystem
  Subsystem C_N_A : Subsystem
  C_L_A : Outport  VectorParamsAs1DForOutWhenUnconnected=off
  C_M_A : Outport  Port=2  VectorParamsAs1DForOutWhenUnconnected=off
  C_N_A : Outport  Port=3  VectorParamsAs1DForOutWhenUnconnected=off
  wires:
  "Subsystem C_M_A "/1(C_M_A) -> C_M_A/1
  "Subsystem C_L_A "/1(C_L_A) -> C_L_A/1
  Subsystem C_N_A/1(C_N_A) -> C_N_A/1
  Mach Number/1 -> "Subsystem C_L_A "/1(Mach Number), "Subsystem C_M_A "/1(Mach Number), Subsystem C_N_A/1(Mach Number)
  alpha_t/1 -> Subsystem C_N_A/2(alpha_t), "Subsystem C_M_A "/2(alpha_t), "Subsystem C_L_A "/2(alpha_t)
  phi_t/1 -> Subsystem C_N_A/3(phi_t), "Subsystem C_M_A "/3(phi_t), "Subsystem C_L_A "/3(phi_t)
  alpha_beta_V/1 -> "Subsystem C_L_A "/4(alpha_beta_V), "Subsystem C_M_A "/4(alpha_beta_V), Subsystem C_N_A/4(alpha_beta_V)
  PQR/1 -> "Subsystem C_M_A "/5(PQR), "Subsystem C_L_A "/5(PQR), Subsystem C_N_A/5(PQR)
  control/1 -> "Subsystem C_M_A "/6(control), "Subsystem C_L_A "/6(control), Subsystem C_N_A/6(control)
  C_X_C_Y_CZ/1 -> "Subsystem C_M_A "/7(C_X_C_Y_C_Z), Subsystem C_N_A/7(C_X_C_Y_C_Z)

== system Missile_Simulink_model/Missile Dynamics/Aerodynamics/Aerodynamic Coefficient/Aerodynamics/Aerodynamic Coef. Translation/Subsystem Aero. Coef. Translation ==
  Mach number : Inport
  alpha_t : Inport  Port=2
  delta_eff : Inport  Port=3
  control : Inport  Port=4
  phi_t : Inport  Port=5
  Subsystem C_X_A : Subsystem
  Subsystem C_Y_A : Subsystem
  Subsystem C_Z_A : Subsystem
  C_X_A : Outport  VectorParamsAs1DForOutWhenUnconnected=off
  C_Y_A : Outport  Port=2  VectorParamsAs1DForOutWhenUnconnected=off
  C_Z_A : Outport  Port=3  VectorParamsAs1DForOutWhenUnconnected=off
  wires:
  Subsystem C_X_A/1(C_X_A) -> C_X_A/1
  Subsystem C_Y_A/1(C_Y_A) -> C_Y_A/1
  Subsystem C_Z_A/1(C_Z_A) -> C_Z_A/1
  Mach number/1 -> Subsystem C_Z_A/1(Mach Number), Subsystem C_Y_A/1(Mach Number), Subsystem C_X_A/1(Mach Number)
  alpha_t/1 -> Subsystem C_Z_A/2(alpha_t), Subsystem C_Y_A/2(alpha_t), Subsystem C_X_A/2(alpha_t)
  delta_eff/1 -> Subsystem C_X_A/3(delta_eff)
  control/1 -> Subsystem C_Z_A/3(control), Subsystem C_Y_A/3(control)
  phi_t/1 -> Subsystem C_Z_A/4(phi_t), Subsystem C_Y_A/4(phi_t)

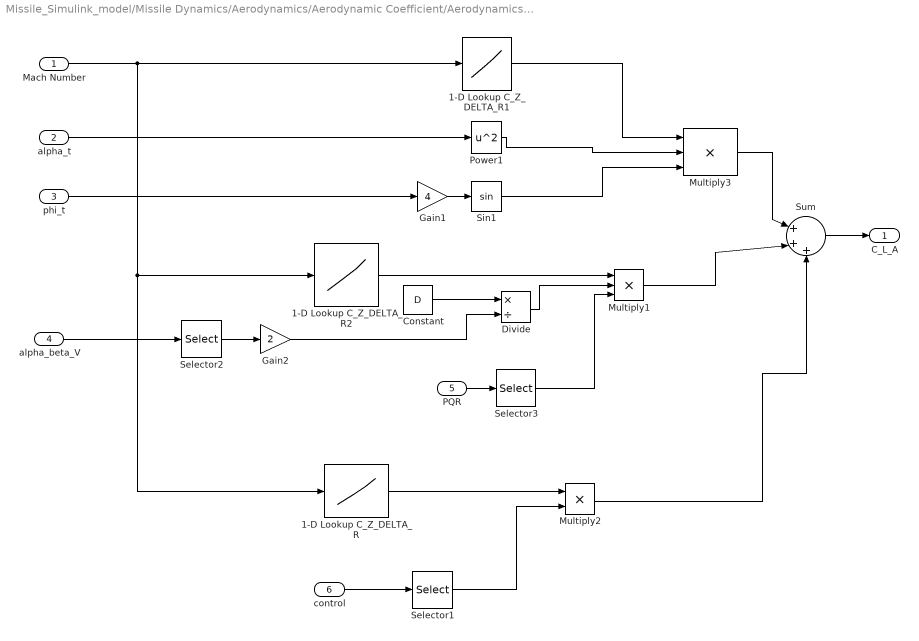
== system Missile_Simulink_model/Missile Dynamics/Aerodynamics/Aerodynamic Coefficient/Aerodynamics/Aerodynamic Coef. Rotation/Subsystem Aero. Coef. Rotation/Subsystem C_L_A  ==
  Mach Number : Inport
  alpha_t : Inport  Port=2
  phi_t : Inport  Port=3
  alpha_beta_V : Inport  Port=4
  PQR : Inport  Port=5
  control : Inport  Port=6
  1-D Lookup C_Z_DELTA_R : Lookup_n-D  NumberOfTableDimensions=1  BreakpointsForDimension1=Tbl_MACH  Table=Tbl_CL_DEL_R  InternalRulePriority=Speed  RndMeth=Simplest  InputSameDT=on
  1-D Lookup C_Z_DELTA_R1 : Lookup_n-D  NumberOfTableDimensions=1  BreakpointsForDimension1=Tbl_MACH  Table=Tbl_CL_ALPHAT  InternalRulePriority=Speed  RndMeth=Simplest  InputSameDT=on
  1-D Lookup C_Z_DELTA_R2 : Lookup_n-D  NumberOfTableDimensions=1  BreakpointsForDimension1=Tbl_MACH  Table=Tbl_CL_P  InternalRulePriority=Speed  RndMeth=Simplest  InputSameDT=on
  Constant : Constant  Value=D
  Divide : Product  Inputs=*/
  Gain1 : Gain  Gain=4
  Gain2 : Gain  Gain=2
  Multiply1 : Product  Inputs=3
  Multiply2 : Product
  Multiply3 : Product  Inputs=3
  Power1 : Math  Operator=square  SignedPower=on  SaturateOnIntegerOverflow=on
  Selector1 : Selector  InputPortWidth=3  IndexOptions=Index vector (dialog)  Indices=[1]  OutputSizes=1
  Selector2 : Selector  InputPortWidth=3  IndexOptions=Index vector (dialog)  Indices=[3]  OutputSizes=1
  Selector3 : Selector  InputPortWidth=3  IndexOptions=Index vector (dialog)  Indices=[1]  OutputSizes=1
  Sin1 : Trigonometry
  Sum : Sum  Inputs=|+++
  C_L_A : Outport  VectorParamsAs1DForOutWhenUnconnected=off
  wires:
  1-D Lookup C_Z_DELTA_R1/1 -> Multiply3/1
  alpha_t/1 -> Power1/1
  Sum/1 -> C_L_A/1
  Mach Number/1 -> 1-D Lookup C_Z_DELTA_R/1, 1-D Lookup C_Z_DELTA_R2/1, 1-D Lookup C_Z_DELTA_R1/1
  1-D Lookup C_Z_DELTA_R2/1 -> Multiply1/1
  1-D Lookup C_Z_DELTA_R/1 -> Multiply2/1
  Multiply2/1 -> Sum/3
  Power1/1 -> Multiply3/2
  Sin1/1 -> Multiply3/3
  phi_t/1 -> Gain1/1
  Gain1/1 -> Sin1/1
  alpha_beta_V/1 -> Selector2/1
  Multiply3/1 -> Sum/1
  Multiply1/1 -> Sum/2
  Constant/1 -> Divide/1
  Selector2/1 -> Gain2/1
  Gain2/1 -> Divide/2
  Divide/1 -> Multiply1/2
  PQR/1 -> Selector3/1
  Selector3/1 -> Multiply1/3
  control/1 -> Selector1/1
  Selector1/1 -> Multiply2/2

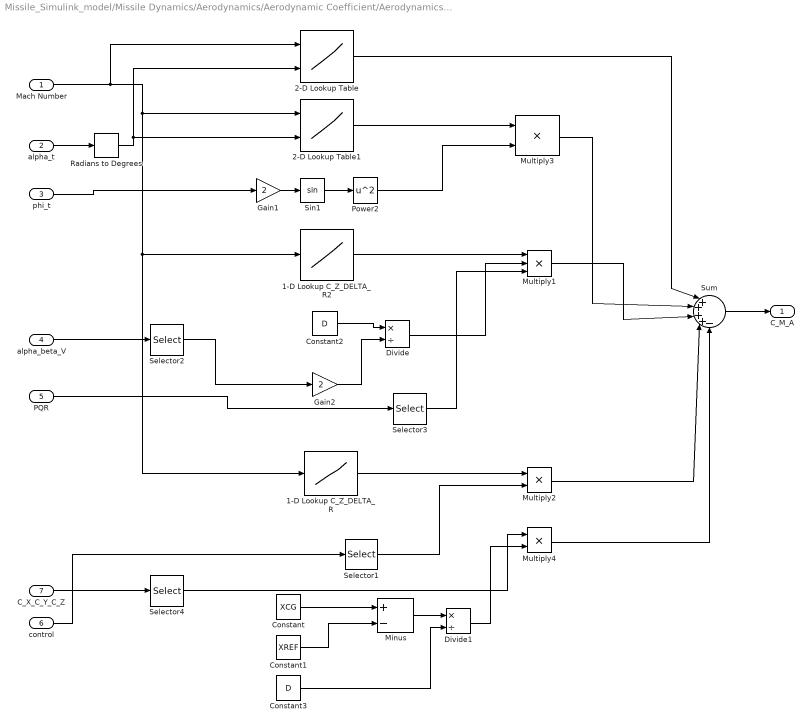
== system Missile_Simulink_model/Missile Dynamics/Aerodynamics/Aerodynamic Coefficient/Aerodynamics/Aerodynamic Coef. Rotation/Subsystem Aero. Coef. Rotation/Subsystem C_M_A  ==
  Mach Number : Inport
  alpha_t : Inport  Port=2
  phi_t : Inport  Port=3
  alpha_beta_V : Inport  Port=4
  PQR : Inport  Port=5
  control : Inport  Port=6
  C_X_C_Y_C_Z : Inport  Port=7
  1-D Lookup C_Z_DELTA_R : Lookup_n-D  NumberOfTableDimensions=1  BreakpointsForDimension1=Tbl_MACH  Table=Tbl_CM_DEL_P  InternalRulePriority=Speed  RndMeth=Simplest  InputSameDT=on
  1-D Lookup C_Z_DELTA_R2 : Lookup_n-D  NumberOfTableDimensions=1  BreakpointsForDimension1=Tbl_MACH  Table=Tbl_CM_Q  DiagnosticForOutOfRangeInput=Warning  InternalRulePriority=Speed  RndMeth=Simplest  InputSameDT=on
  2-D Lookup Table : Lookup_n-D  BreakpointsForDimension1=Tbl_MACH  BreakpointsForDimension2=Tbl_ALPHAT  Table=Tbl_CM_0  DiagnosticForOutOfRangeInput=Warning  InternalRulePriority=Speed  RndMeth=Simplest  InputSameDT=on
      settings: InputPortMap=u0,u1
  2-D Lookup Table1 : Lookup_n-D  BreakpointsForDimension1=Tbl_MACH  BreakpointsForDimension2=Tbl_ALPHAT  Table=Tbl_CM_PHIT  InternalRulePriority=Speed  RndMeth=Simplest  InputSameDT=on
      settings: InputPortMap=u0,u1
  Constant : Constant  Value=XCG
  Constant1 : Constant  Value=XREF
  Constant2 : Constant  Value=D
  Constant3 : Constant  Value=D
  Divide : Product  Inputs=*/
  Divide1 : Product  Inputs=*/
  Gain1 : Gain  Gain=2
  Gain2 : Gain  Gain=2
  Minus : Sum  Inputs=+-
  Multiply1 : Product  Inputs=3
  Multiply2 : Product
  Multiply3 : Product
  Multiply4 : Product
  Power2 : Math  Operator=square  SignedPower=on  SaturateOnIntegerOverflow=on
  Radians to Degrees : simulink_extras/Transformations/Radians to Degrees
  Selector1 : Selector  InputPortWidth=3  IndexOptions=Index vector (dialog)  Indices=[2]  OutputSizes=1
  Selector2 : Selector  InputPortWidth=3  IndexOptions=Index vector (dialog)  Indices=[3]  OutputSizes=1
  Selector3 : Selector  InputPortWidth=3  IndexOptions=Index vector (dialog)  Indices=[2]  OutputSizes=1
  Selector4 : Selector  InputPortWidth=3  IndexOptions=Index vector (dialog)  Indices=[3]  OutputSizes=1
  Sin1 : Trigonometry
  Sum : Sum  Inputs=|++++-
  C_M_A : Outport  VectorParamsAs1DForOutWhenUnconnected=off
  wires:
  2-D Lookup Table/1 -> Sum/1
  Mach Number/1 -> 2-D Lookup Table/1, 2-D Lookup Table1/1, 1-D Lookup C_Z_DELTA_R/1, 1-D Lookup C_Z_DELTA_R2/1
  1-D Lookup C_Z_DELTA_R2/1 -> Multiply1/1
  1-D Lookup C_Z_DELTA_R/1 -> Multiply2/1
  Multiply2/1 -> Sum/4
  Sin1/1 -> Power2/1
  phi_t/1 -> Gain1/1
  Gain1/1 -> Sin1/1
  alpha_beta_V/1 -> Selector2/1
  Selector2/1 -> Gain2/1
  Gain2/1 -> Divide/2
  Divide/1 -> Multiply1/2
  PQR/1 -> Selector3/1
  Selector3/1 -> Multiply1/3
  control/1 -> Selector1/1
  Selector1/1 -> Multiply2/2
  2-D Lookup Table1/1 -> Multiply3/1
  Power2/1 -> Multiply3/2
  C_X_C_Y_C_Z/1 -> Selector4/1
  Constant/1 -> Minus/1
  Constant1/1 -> Minus/2
  Constant2/1 -> Divide/1
  Minus/1 -> Divide1/1
  Constant3/1 -> Divide1/2
  Selector4/1 -> Multiply4/1
  Divide1/1 -> Multiply4/2
  Multiply4/1 -> Sum/5
  Multiply1/1 -> Sum/3
  Multiply3/1 -> Sum/2
  alpha_t/1 -> Radians to Degrees/1
  Radians to Degrees/1 -> 2-D Lookup Table1/2, 2-D Lookup Table/2
  Sum/1 -> C_M_A/1

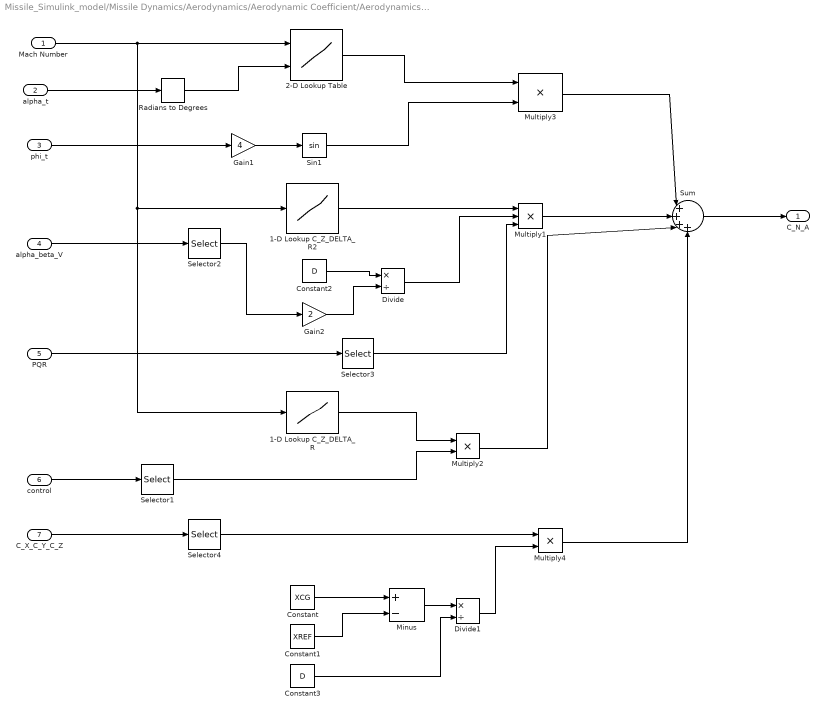
== system Missile_Simulink_model/Missile Dynamics/Aerodynamics/Aerodynamic Coefficient/Aerodynamics/Aerodynamic Coef. Rotation/Subsystem Aero. Coef. Rotation/Subsystem C_N_A ==
  Mach Number : Inport
  alpha_t : Inport  Port=2
  phi_t : Inport  Port=3
  alpha_beta_V : Inport  Port=4
  PQR : Inport  Port=5
  control : Inport  Port=6
  C_X_C_Y_C_Z : Inport  Port=7
  1-D Lookup C_Z_DELTA_R : Lookup_n-D  NumberOfTableDimensions=1  BreakpointsForDimension1=Tbl_MACH  Table=Tbl_CN_DEL_Y  InternalRulePriority=Speed  RndMeth=Simplest  InputSameDT=on
  1-D Lookup C_Z_DELTA_R2 : Lookup_n-D  NumberOfTableDimensions=1  BreakpointsForDimension1=Tbl_MACH  Table=Tbl_CN_R  InternalRulePriority=Speed  RndMeth=Simplest  InputSameDT=on
  2-D Lookup Table : Lookup_n-D  BreakpointsForDimension1=Tbl_MACH  BreakpointsForDimension2=Tbl_ALPHAT  Table=Tbl_CN_PHIT  InternalRulePriority=Speed  RndMeth=Simplest  InputSameDT=on
      settings: InputPortMap=u0,u1
  Constant : Constant  Value=XCG
  Constant1 : Constant  Value=XREF
  Constant2 : Constant  Value=D
  Constant3 : Constant  Value=D
  Divide : Product  Inputs=*/
  Divide1 : Product  Inputs=*/
  Gain1 : Gain  Gain=4
  Gain2 : Gain  Gain=2
  Minus : Sum  Inputs=+-
  Multiply1 : Product  Inputs=3
  Multiply2 : Product
  Multiply3 : Product
  Multiply4 : Product
  Radians to Degrees : simulink_extras/Transformations/Radians to Degrees
  Selector1 : Selector  InputPortWidth=3  IndexOptions=Index vector (dialog)  Indices=[3]  OutputSizes=1
  Selector2 : Selector  InputPortWidth=3  IndexOptions=Index vector (dialog)  Indices=[3]  OutputSizes=1
  Selector3 : Selector  InputPortWidth=3  IndexOptions=Index vector (dialog)  Indices=[3]  OutputSizes=1
  Selector4 : Selector  InputPortWidth=3  IndexOptions=Index vector (dialog)  Indices=[2]  OutputSizes=1
  Sin1 : Trigonometry
  Sum : Sum  Inputs=|++++
  C_N_A : Outport  VectorParamsAs1DForOutWhenUnconnected=off
  wires:
  2-D Lookup Table/1 -> Multiply3/1
  alpha_t/1 -> Radians to Degrees/1
  Sum/1 -> C_N_A/1
  Mach Number/1 -> 2-D Lookup Table/1, 1-D Lookup C_Z_DELTA_R/1, 1-D Lookup C_Z_DELTA_R2/1
  1-D Lookup C_Z_DELTA_R2/1 -> Multiply1/1
  1-D Lookup C_Z_DELTA_R/1 -> Multiply2/1
  Multiply2/1 -> Sum/3
  Sin1/1 -> Multiply3/2
  phi_t/1 -> Gain1/1
  Gain1/1 -> Sin1/1
  alpha_beta_V/1 -> Selector2/1
  Selector2/1 -> Gain2/1
  Divide/1 -> Multiply1/2
  PQR/1 -> Selector3/1
  Selector3/1 -> Multiply1/3
  control/1 -> Selector1/1
  Selector1/1 -> Multiply2/2
  C_X_C_Y_C_Z/1 -> Selector4/1
  Constant/1 -> Minus/1
  Constant1/1 -> Minus/2
  Constant2/1 -> Divide/1
  Minus/1 -> Divide1/1
  Constant3/1 -> Divide1/2
  Selector4/1 -> Multiply4/1
  Divide1/1 -> Multiply4/2
  Multiply4/1 -> Sum/4
  Multiply1/1 -> Sum/2
  Multiply3/1 -> Sum/1
  Radians to Degrees/1 -> 2-D Lookup Table/2
  Gain2/1 -> Divide/2

== system Missile_Simulink_model/Missile Dynamics/Aerodynamics/Aerodynamic Coefficient/Aerodynamics/Aerodynamic Coef. Translation/Subsystem Aero. Coef. Translation/Subsystem C_X_A ==
  Mach Number : Inport
  alpha_t : Inport  Port=2
  delta_eff : Inport  Port=3
  1-D Lookup C_X_0 : Lookup_n-D  NumberOfTableDimensions=1  BreakpointsForDimension1=Tbl_MACH  Table=Tbl_CX_0  DiagnosticForOutOfRangeInput=Error  InternalRulePriority=Speed  RndMeth=Simplest  InputSameDT=on
  1-D Lookup C_X_ALPHA_T : Lookup_n-D  NumberOfTableDimensions=1  BreakpointsForDimension1=Tbl_MACH  BeginIndexSearchUsingPreviousIndexResult=on  Table=Tbl_CX_ALPHAT  DiagnosticForOutOfRangeInput=Error  InternalRulePriority=Speed  RndMeth=Simplest  InputSameDT=on
  1-D Lookup C_X_DELTA_EFF : Lookup_n-D  NumberOfTableDimensions=1  BreakpointsForDimension1=Tbl_MACH  Table=Tbl_CX_DEL_EFF  DiagnosticForOutOfRangeInput=Error  InternalRulePriority=Speed  RndMeth=Simplest  InputSameDT=on
  Multiply : Product
  Multiply1 : Product
  Square : Math  Operator=square  SignedPower=on  SaturateOnIntegerOverflow=on
  Sum : Sum  Inputs=|+++
  C_X_A : Outport  VectorParamsAs1DForOutWhenUnconnected=off
  wires:
  Multiply/1 -> Sum/2
  Multiply1/1 -> Sum/3
  1-D Lookup C_X_DELTA_EFF/1 -> Multiply1/1
  1-D Lookup C_X_ALPHA_T/1 -> Multiply/1
  1-D Lookup C_X_0/1 -> Sum/1
  Mach Number/1 -> 1-D Lookup C_X_DELTA_EFF/1, 1-D Lookup C_X_ALPHA_T/1, 1-D Lookup C_X_0/1
  Sum/1 -> C_X_A/1
  alpha_t/1 -> Multiply/2
  delta_eff/1 -> Square/1
  Square/1 -> Multiply1/2
